simulink model "ArduinoGPIO2"  (R2024a)
settings: Solver=FixedStepAuto  StartTime=0.0  StopTime=60  RelTol=1e-3  EnableMultiTasking=on
values from neighbouring files (symbols this model uses):
  L_gain = acker(ssmodel_A',ssmodel_C',p_observer)'    [param_init.m]
  max_dc = (1.5e-3/(1/pwm_freq))*255    [param_init.m]
  max_dc_init = (2e-3/(1/pwm_freq))*255    [param_init.m]
  min_dc = (1e-3/(1/pwm_freq))*255    [param_init.m]
  min_dc_init = (1e-3/(1/pwm_freq))*255    [param_init.m]
  pot_gain = single(180/516)    [param_init.m]
  pot_offset = single(512)    [param_init.m]
  pwm_gain = (max_dc-min_dc)    [param_init.m]
  R = round(conv(F_RST,Rp_RST),3)    [param_init.m]
  r0_meq = (1+p1+p2)/(b1+b2)    [ModelPendulum.m]    (also in param_init.m)
  r1_meq = a1*r0_meq    [ModelPendulum.m]    (also in param_init.m)
  r2_meq = a2*r0_meq    [ModelPendulum.m]    (also in param_init.m)
  s1_meq = r0_meq*b2-p2    [ModelPendulum.m]    (also in param_init.m)
  ssmodel_A = [0 1; -(model.M*model.g*model.x)/model.J -model.b/model.J]    [param_init.m]
  ssmodel_B = [0 model.gain/model.J]'    [param_init.m]
  ssmodel_C = [1 0]    [param_init.m]
  T = P_RST/sum(num)    [param_init.m]
  Ts = 5e-2    (= 0.05)    [param_init.m]
  Ts_a = 5e-2    (= 0.05)    [param_init.m]
undefined symbols (not defined in the file or in its folder): control, den_mf_track, DiscIntNeverNeededParam, K_controller, K_controller2, model, num_mf_track
libraries: arduinolib x3, simulink x1
settings Model: ExtModeTrigDuration=2  Creator=Douglas  LastModifiedBy=Douglas
settings SolverCC: AutoInsertRateTranBlk=on
settings OptimizationCC: EnhancedBackFolding=on  PassReuseOutputArgsAs=Individual arguments  ZeroExternalMemoryAtStartup=off  ZeroInternalMemoryAtStartup=off  MaxStackSize=64  OptimizeBlockOrder=speed  DifferentSizesBufferReuse=on  OptimizationCustomize=off  EfficientTunableParamExpr=on
settings DebuggingCC: ParameterTunabilityLossMsg=error
settings HardwareCC: ProdBitPerInt=16  ProdBitPerPointer=16  ProdBitPerSizeT=16  ProdBitPerPtrDiffT=16  ProdLargestAtomicFloat=None  ProdWordSize=8  ProdHWDeviceType=Atmel->AVR
settings ModelReferenceCC: PropagateVarSize=During execution
settings SFSimCC: MATLABDynamicMemAlloc=off
settings RTWCC: Description=Embedded Coder  SystemTargetFile=ert.tlc  HardwareBoard=Arduino Uno  TemplateMakefile=ert_default_tmf  Toolchain=Arduino AVR  BuildConfiguration=Faster Runs
settings CodeAppCC: ForceParamTrailComments=on  IgnoreCustomStorageClasses=off  OperatorAnnotations=on  SimulinkDataObjDesc=on  SFDataObjDesc=on  InsertBlockDesc=on
settings ERTTargetCC: SupportContinuousTime=on  SupportVariableSizeSignals=on  ExtModeTransport=3  ExtModeStaticAlloc=on  ExtModeAutomaticAllocSize=off  ExtModeStaticAllocSize=250  ExtModeMexFile=ext_xcp  ExtModeIntrfLevel=Level2 - Open

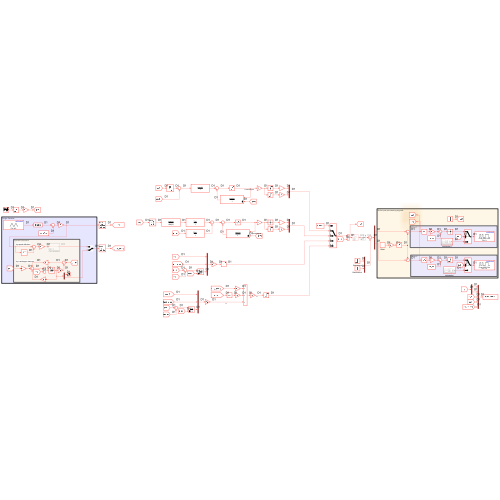
[thumbnail: Simulink's stored preview of the top-level diagram]
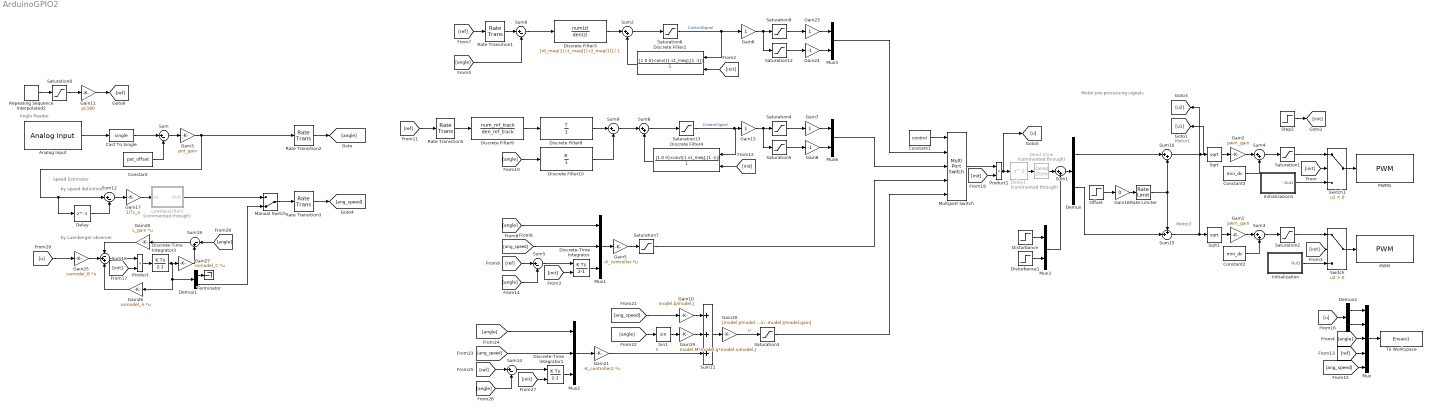
== system ArduinoGPIO2 ==
  note: Motor pre-processing signals
  note: by speed definition
  note: Speed Estimator
  note: Motor2
  note: Motor1
  note: Angle Reader
  note: by Luenberger observer
  Analog Input : arduinolib/Analog Input  pinNumber=0  ReadResultsOnly=off  ConversionTriggerSource=Software  ExternalTriggerType=uint32( 0 )  OutputDataType=uint16  EnableConversionCompleteNotify=off  EnableOuputStatus=off  SampleTime=Ts_a  blockPlatform=arduino
  Cast To Single : DataTypeConversion  OutDataTypeStr=single  SaturateOnIntegerOverflow=off  RndMeth=Floor
  Constant : Constant  Value=pot_offset  OutDataTypeStr=single  SampleTime=Ts_a
  Constant1 : Constant  Value=control  SampleTime=Ts
  Constant2 : Constant  Value=min_dc  OutDataTypeStr=single  SampleTime=Ts
  Constant3 : Constant  Value=min_dc  OutDataTypeStr=single  SampleTime=Ts
  Dead Zone : DeadZone  Commented=through  LowerValue=0  UpperValue=0.1
  Delay : Delay  DelayLength=1
  Delay1 : Delay  Commented=through
  Demux : Demux  Outputs=2
  Demux1 : Demux  Outputs=2
  Demux2 : Demux  Outputs=2
  Discrete Filter10 : DiscreteFilter  Numerator=R  Denominator=1
  Discrete Filter2 : DiscreteFilter  Numerator=[1 0 0]-conv([1 s1_meq],[1 -1])  Denominator=1  ExternalReset=Rising
      settings: InputPortMap=u0,r7
  Discrete Filter3 : DiscreteFilter  Numerator=[r0_meq(1) r1_meq(1) r2_meq(1)]  Denominator=1
  Discrete Filter4 : DiscreteFilter  Numerator=[1 0 0]-conv([1 s1_meq],[1 -1])  Denominator=1  ExternalReset=Rising
      settings: InputPortMap=u0,r7
  Discrete Filter8 : DiscreteFilter  Numerator=T  Denominator=1
  Discrete Filter9 : DiscreteFilter  Numerator=num_mf_track  Denominator=den_mf_track
  Discrete-Time Integrator : DiscreteIntegrator  ExternalReset=rising  SampleTime=-1  ICPrevOutput=DiscIntNeverNeededParam  ICPrevScaledInput=DiscIntNeverNeededParam
  Discrete-Time Integrator1 : DiscreteIntegrator  ExternalReset=rising  SampleTime=-1  ICPrevOutput=DiscIntNeverNeededParam  ICPrevScaledInput=DiscIntNeverNeededParam
  Discrete-Time Integrator3 : DiscreteIntegrator  SampleTime=-1  ICPrevOutput=DiscIntNeverNeededParam  ICPrevScaledInput=DiscIntNeverNeededParam
  Disturbance : Step  Time=5+15  After=0.04  SampleTime=Ts
  Disturbance1 : Step  Time=20+15  After=0.04  SampleTime=Ts
  Gain1 : Gain  Gain=pwm_gain  ParamDataTypeStr=single  OutDataTypeStr=Inherit: Inherit via back propagation
  Gain10 : Gain  Gain=model.b/model.J
  Gain11 : Gain  Gain=pi/180
  Gain{6..7,15,23} (4 alike) : Gain
  Gain16 : Gain  Gain=0
  Gain17 : Gain  Gain=1/Ts_a
  Gain19 : Gain  Gain=model.M*model.g*model.x/model.J
  Gain2 : Gain  Gain=pwm_gain  OutDataTypeStr=single
  Gain20 : Gain  Gain=[model.J/model.gain -model.J/model.gain]
  Gain21 : Gain  Gain=-K_controller2  Multiplication=Matrix(K*u)
  Gain24 : Gain  Gain=-1
  Gain25 : Gain  Gain=ssmodel_B  Multiplication=Matrix(K*u)  OutDataTypeStr=single
  Gain26 : Gain  Gain=ssmodel_A  Multiplication=Matrix(K*u)
  Gain27 : Gain  Gain=ssmodel_C  Multiplication=Matrix(K*u)
  Gain28 : Gain  Gain=L_gain  Multiplication=Matrix(K*u)
  Gain3 : Gain  Gain=pot_gain  OutDataTypeStr=single
  Gain5 : Gain  Gain=-K_controller  Multiplication=Matrix(K*u)
  Gain8 : Gain  Gain=-1
  Initialization : Subsystem
  Initialization1 : Subsystem
  LowPassFilter1 : Subsystem  Commented=through  mask{tau=Ts_a, Ts=Ts_a}
      mask prompts: tau "Time constant"; Ts "Sample Time"
      mask DialogControl DescGroupVar Prompt: Discrete LP Filter
  Manual Switch : ManualSwitch  CurrentSetting=0
  Multiport Switch : MultiPortSwitch  Inputs=4  SaturateOnIntegerOverflow=off  InputSameDT=off
  Mux : Mux  Inputs=5
  Mux1 : Mux  Inputs=3
  Mux2 : Mux  Inputs=3
  Mux3 : Mux  Inputs=2
  Mux5 : Mux  Inputs=2
  Mux6 : Mux  Inputs=2
  Offset : Step  Time=15  After=0.01  OutDataTypeStr=single  SampleTime=Ts
  PWM : arduinolib/PWM  pinNumber=motor2  frequencyType=Specify  desiredFrequency=pwm_freq  achievableFrequency=490.1961
  PWM1 : arduinolib/PWM  pinNumber=motor1  frequencyType=Specify  desiredFrequency=pwm_freq  achievableFrequency=490.1961
  Product : Product
  Product1 : Product
  Rate Limiter : RateLimiter  SampleTimeMode=inherited
  Rate Transition1 : RateTransition
  Rate Transition2 : RateTransition  OutPortSampleTime=Ts
  Rate Transition3 : RateTransition  OutPortSampleTime=Ts
  Rate Transition5 : RateTransition
  Repeating Sequence Interpolated2 : simulink/Sources/Repeating Sequence Interpolated  OutValues=[0 0 20 20 -45 -45 60 60].'  TimeValues=[0 15 15+Ts 30 30+Ts 45 45+Ts 60].'  LookUpMeth=Interpolation-Use End Values  tsamp=Ts  OutMin=[]  OutMax=[]  OutDataTypeStr=single  OutputDataTypeScalingMode=single  OutDataType=fixdt(0,8)  OutScaling=2^-10
  Saturation1 : Saturate  UpperLimit=max_dc  LowerLimit=min_dc  OutDataTypeStr=single
  Saturation12 : Saturate  UpperLimit=0  LowerLimit=-1
  Saturation13 : Saturate  UpperLimit=1  LowerLimit=-1
  Saturation2 : Saturate  UpperLimit=max_dc  LowerLimit=min_dc
  Saturation{3..4,7,9} (4 alike) : Saturate  UpperLimit=1  LowerLimit=0
  Saturation5 : Saturate  UpperLimit=0  LowerLimit=-1
  Saturation6 : Saturate  UpperLimit=1  LowerLimit=-1
  Saturation8 : Saturate  UpperLimit=140  LowerLimit=-140
  Sin1 : Trigonometry
  Sqrt : Sqrt  OutputSignalType=real
  Sqrt1 : Sqrt  OutputSignalType=real
  Step2 : Step  Time=15  OutDataTypeStr=single  SampleTime=Ts
  Sum{,5..6,12,14} (5 alike) : Sum  Inputs=|+-
  Sum1 : Sum  Inputs=|++
  Sum10 : Sum  Inputs=|++
  Sum11 : Sum  Inputs=+++
  Sum15 : Sum  Inputs=++|
  Sum18 : Sum  Inputs=-++
  Sum19 : Sum  Inputs=|-+
  Sum2 : Sum  Inputs=|++  OutDataTypeStr=single
  Sum3 : Sum  Inputs=|++  OutDataTypeStr=Inherit: Same as first input
  Sum4 : Sum  Inputs=|++  OutDataTypeStr=Inherit: Same as first input
  Sum8 : Sum  Inputs=|++  OutDataTypeStr=single
  Sum9 : Sum  Inputs=|+-  OutDataTypeStr=Inherit: Inherit via back propagation
  Switch : Switch  Criteria=u2 > Threshold  SaturateOnIntegerOverflow=off  InputSameDT=off
  Switch1 : Switch  Criteria=u2 > Threshold  SaturateOnIntegerOverflow=off  InputSameDT=off
  Terminator : Terminator
  To Workspace : ToWorkspace  VariableName=Ensaio1  SaveFormat=Structure With Time  SampleTime=Ts
  wires:
  Constant/1 -> Sum/2
  Constant2/1 -> Sum3/2
  Initialization/1(Out1) -> Switch/3
  Initialization1/1(Out1) -> Switch1/3
  Saturation1/1 -> Switch1/1
  [init] -> Switch/2
  Sum/1 -> Gain3/1
  Gain1/1 -> Sum3/1
  Constant3/1 -> Sum4/2
  Analog Input/1 -> Cast To Single/1
  Sum4/1 -> Saturation1/1
  Saturation2/1 -> Switch/1
  Sum3/1 -> Saturation2/1
  Gain2/1 -> Sum4/1
  Step2/1 -> [init]
  [init] -> Switch1/2
  Cast To Single/1 -> Sum/1
  Switch/1 -> PWM/1
  Switch1/1 -> PWM1/1
  Sum10/1 -> Sqrt/1, [u1]
  Sum15/1 -> [u2], Sqrt1/1
  Demux2/1 -> Mux/1
  Demux2/2 -> Mux/2
  [angle] -> Mux/3
  Mux/1 -> To Workspace/1
  Sqrt/1 -> Gain2/1
  Sqrt1/1 -> Gain1/1
  Offset/1 -> Gain16/1
  Gain16/1 -> Rate Limiter/1
  Rate Limiter/1 -> Sum15/1, Sum10/2
  [ref] -> Mux/4
  Delay/1 -> Sum12/2
  Sum12/1 -> Gain17/1
  [ang_speed] -> Mux/5
  Manual Switch/1 -> Rate Transition3/1
  Gain17/1 -> LowPassFilter1/1(In1)
  LowPassFilter1/1(Out1) -> Manual Switch/1
  Rate Transition2/1 -> [angle]
  Rate Transition3/1 -> [ang_speed]
  Gain3/1 -> Rate Transition2/1, Delay/1, Sum12/1
  Sum18/1 -> Product/1
  Sum19/1 -> Gain28/1
  Gain25/1 -> Sum18/2
  [angle] -> Sum19/1
  Discrete-Time Integrator3/1 -> Gain26/1, Demux1/1, Gain27/1
  Gain27/1 -> Sum19/2
  Gain26/1 -> Sum18/3
  Demux1/1 -> Terminator/1
  Gain28/1 -> Sum18/1
  Demux1/2 -> Manual Switch/2
  [u] -> Gain25/1
  Demux/2 -> Sum15/2
  Saturation9/1 -> Gain23/1
  Rate Transition1/1 -> Sum6/1
  [ref] -> Rate Transition1/1
  Saturation8/1 -> Gain11/1
  Discrete Filter9/1 -> Discrete Filter8/1
  [angle] -> Sum6/2
  Sum6/1 -> Discrete Filter3/1
  Discrete Filter3/1 -> Sum2/1
  Discrete Filter4/1 -> Sum8/2
  Sum9/1 -> Sum8/1
  Saturation13/1 -> Discrete Filter4/1, Gain15/1  "ControlSignal"
  [angle] -> Mux2/1
  Mux2/1 -> Gain21/1
  Gain7/1 -> Mux6/1
  Constant1/1 -> Multiport Switch/1
  Disturbance1/1 -> Mux3/2
  Sum8/1 -> Saturation13/1
  Discrete Filter2/1 -> Sum2/2
  [init] -> Discrete-Time Integrator1/2
  Gain20/1 -> Saturation3/1  "U"
  Mux6/1 -> Multiport Switch/3
  [ref] -> Sum14/1
  Repeating Sequence Interpolated2/1 -> Saturation8/1
  Mux5/1 -> Multiport Switch/2
  Disturbance/1 -> Mux3/1
  Mux3/1 -> Sum1/2
  Saturation4/1 -> Gain7/1
  [angle] -> Discrete Filter10/1
  Gain8/1 -> Mux6/2
  Rate Transition5/1 -> Discrete Filter9/1
  Gain23/1 -> Mux5/1
  Saturation12/1 -> Gain24/1
  Discrete-Time Integrator/1 -> Mux1/3
  Saturation5/1 -> Gain8/1
  Sum11/1 -> Gain20/1
  Product1/1 -> [u], Delay1/1
  [ref] -> Sum5/1
  [angle] -> Sum14/2
  Sin1/1 -> Gain19/1
  Discrete Filter10/1 -> Sum9/2
  Gain11/1 -> [ref]
  [ang_speed] -> Mux1/2
  Mux1/1 -> Gain5/1
  Discrete Filter8/1 -> Sum9/1
  [init] -> Discrete Filter4/2
  [ref] -> Rate Transition5/1
  Saturation7/1 -> Multiport Switch/4
  Sum2/1 -> Saturation6/1
  Discrete-Time Integrator1/1 -> Mux2/3
  Gain21/1 -> Sum11/3  "U"
  Gain6/1 -> Saturation12/1, Saturation9/1
  Saturation6/1 -> Gain6/1, Discrete Filter2/1  "ControlSignal"
  Gain10/1 -> Sum11/1
  Gain24/1 -> Mux5/2
  [ang_speed] -> Gain10/1
  [angle] -> Sum5/2
  [angle] -> Sin1/1
  [ang_speed] -> Mux2/2
  Gain15/1 -> Saturation4/1, Saturation5/1
  [angle] -> Mux1/1
  Gain19/1 -> Sum11/2
  Saturation3/1 -> Multiport Switch/5
  Sum14/1 -> Discrete-Time Integrator1/1
  Gain5/1 -> Saturation7/1
  Sum5/1 -> Discrete-Time Integrator/1
  Demux/1 -> Sum10/1
  Sum1/1 -> Demux/1
  [u] -> Demux2/1
  [init] -> Discrete Filter2/2
  [init] -> Discrete-Time Integrator/2
  [init] -> Product/2
  Product/1 -> Discrete-Time Integrator3/1
  [init] -> Product1/2
  Multiport Switch/1 -> Product1/1
  Delay1/1 -> Dead Zone/1
  Dead Zone/1 -> Sum1/1

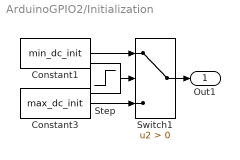
== system ArduinoGPIO2/Initialization ==
  Constant1 : Constant  Value=min_dc_init  OutDataTypeStr=single  SampleTime=Ts
  Constant3 : Constant  Value=max_dc_init  OutDataTypeStr=single  SampleTime=Ts
  Step : Step  Time=2  OutDataTypeStr=single  SampleTime=Ts
  Switch1 : Switch  Criteria=u2 > Threshold  SaturateOnIntegerOverflow=off  InputSameDT=off
  Out1 : Outport
  wires:
  Step/1 -> Switch1/2
  Switch1/1 -> Out1/1
  Constant3/1 -> Switch1/3
  Constant1/1 -> Switch1/1

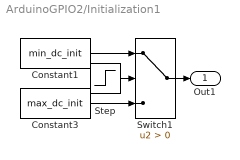
== system ArduinoGPIO2/Initialization1 ==
  Constant1 : Constant  Value=min_dc_init  OutDataTypeStr=single  SampleTime=Ts
  Constant3 : Constant  Value=max_dc_init  OutDataTypeStr=single  SampleTime=Ts
  Step : Step  Time=2  OutDataTypeStr=single  SampleTime=Ts
  Switch1 : Switch  Criteria=u2 > Threshold  SaturateOnIntegerOverflow=off  InputSameDT=off
  Out1 : Outport
  wires:
  Constant1/1 -> Switch1/1
  Constant3/1 -> Switch1/3
  Switch1/1 -> Out1/1
  Step/1 -> Switch1/2

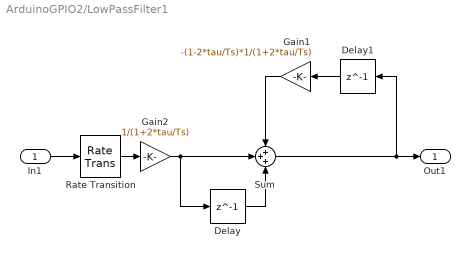
== system ArduinoGPIO2/LowPassFilter1 ==
  In1 : Inport
  Delay : Delay  DelayLength=1
  Delay1 : Delay  DelayLength=1
  Gain1 : Gain  Gain=-(1-2*tau/Ts)*1/(1+2*tau/Ts)  OutDataTypeStr=single
  Gain2 : Gain  Gain=1/(1+2*tau/Ts)  OutDataTypeStr=single
  Rate Transition : RateTransition  OutPortSampleTime=Ts
  Sum : Sum  Inputs=+++
  Out1 : Outport
  wires:
  Sum/1 -> Out1/1, Delay1/1
  Delay1/1 -> Gain1/1
  Delay/1 -> Sum/3
  In1/1 -> Rate Transition/1
  Rate Transition/1 -> Gain2/1
  Gain2/1 -> Sum/2, Delay/1
  Gain1/1 -> Sum/1
